simulink model "lab_model"  (Simulink 9.2)
settings: Solver=ode45  StartTime=0.0  StopTime=1  RelTol=1e-3  EnableMultiTasking=on
values from neighbouring files (symbols this model uses):
  A0 = 2.5    [lab_vars.m]
  J = Jco+Jm    (= 10.2)    [lab_vars.m]
  Kcur_fdb = round(kcs*kadc)    [lab_vars.m]
  kcur_i = 5    [lab_vars.m]
  kcur_p = 10    [lab_vars.m]
  Ke = Km    (= 5)    [lab_vars.m]
  Km = 5    [lab_vars.m]
  Kpwc = Un/Uc    (= 2.5)    [lab_vars.m]
  Kspd_fdb = round(kps_int*Ts,1)    [lab_vars.m]
  kspd_p = 10    [lab_vars.m]
  R = 5    [lab_vars.m]
  Te = 0.0005    [lab_vars.m]
  Tpwc = 0.002    [lab_vars.m]
  W0 = 100    [lab_vars.m]
settings Model: Creator=Student  LastModifiedBy=murad
settings DataIOCC: LimitDataPoints=off  SaveFormat=StructureWithTime
settings DebuggingCC: UnderspecifiedInitializationDetection=Simplified  MergeDetectMultiDrivingBlocksExec=error  StateNameClashWarn=none
settings HardwareCC: ProdIntDivRoundTo=Zero  ProdEndianess=LittleEndian  ProdHWDeviceType=Specified

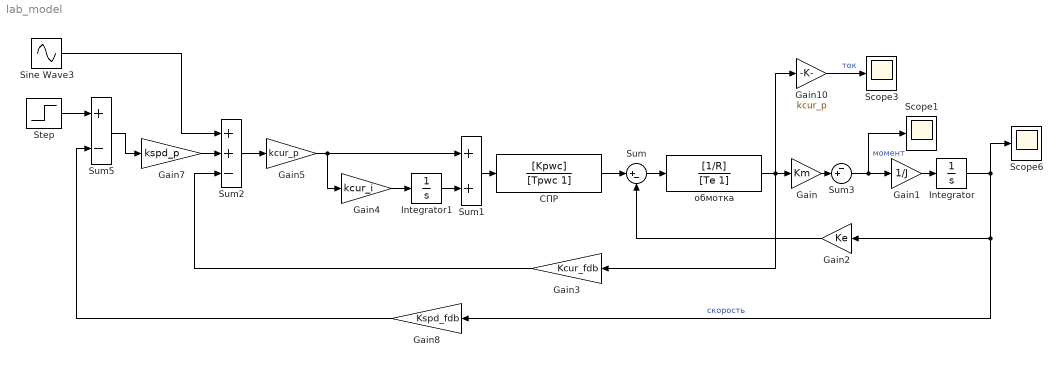
== system lab_model ==
  Gain : Gain  Gain=Km
  Gain1 : Gain  Gain=1/J
  Gain10 : Gain  Gain=kcur_p
  Gain2 : Gain  Gain=Ke
  Gain3 : Gain  Gain=Kcur_fdb
  Gain4 : Gain  Gain=kcur_i
  Gain5 : Gain  Gain=kcur_p
  Gain7 : Gain  Gain=kspd_p
  Gain8 : Gain  Gain=Kspd_fdb
  Integrator : Integrator
  Integrator1 : Integrator
  Scope1 : Scope
  Scope3 : Scope
  Scope6 : Scope
  Sine Wave3 : Sin  Amplitude=A0*1.2  Frequency=W0  SampleTime=0
  Step : Step  Time=0  After=A0  SampleTime=0
  Sum : Sum  Inputs=|+-
  Sum1 : Sum
  Sum2 : Sum  Inputs=++-
  Sum3 : Sum  Inputs=-+|
  Sum5 : Sum  Inputs=+-
  СПР : TransferFcn  Numerator=[Kpwc]  Denominator=[Tpwc 1]
  обмотка : TransferFcn  Numerator=[1/R]  Denominator=[Te 1]
  wires:
  обмотка/1 -> Gain10/1, Gain3/1, Gain/1
  Gain1/1 -> Integrator/1
  Sum/1 -> обмотка/1
  Gain2/1 -> Sum/2
  Integrator/1 -> Scope6/1, Gain8/1, Gain2/1  "скорость"
  СПР/1 -> Sum/1
  Sum1/1 -> СПР/1
  Gain4/1 -> Integrator1/1
  Gain5/1 -> Gain4/1, Sum1/1
  Sum2/1 -> Gain5/1
  Gain3/1 -> Sum2/3
  Gain/1 -> Sum3/2
  Sum3/1 -> Scope1/1, Gain1/1  "момент"
  Sum5/1 -> Gain7/1
  Gain8/1 -> Sum5/2
  Gain7/1 -> Sum2/2
  Step/1 -> Sum5/1
  Integrator1/1 -> Sum1/2
  Gain10/1 -> Scope3/1  "ток"
  Sine Wave3/1 -> Sum2/1
